simulink model "Practica1"  (R2024a)
settings: Solver=VariableStepAuto  StartTime=0.0  StopTime=10  RelTol=1e-3
InitFcn:
  | m1=0.2;
  | I1=0.3;
  | m2=0.1;
  | I2=0.25;
  | g=9.81;
settings Model: Creator=Becho  LastModifiedBy=Becho

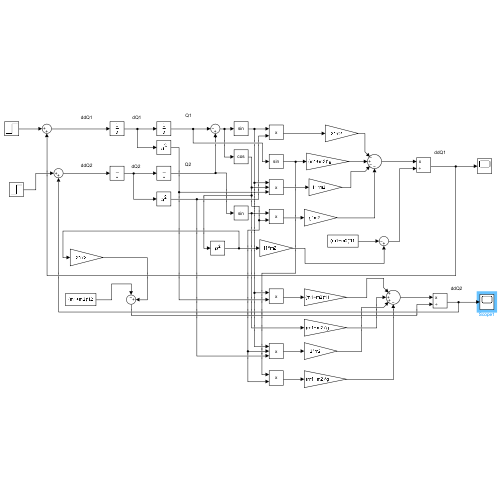
[thumbnail: Simulink's stored preview of the top-level diagram]
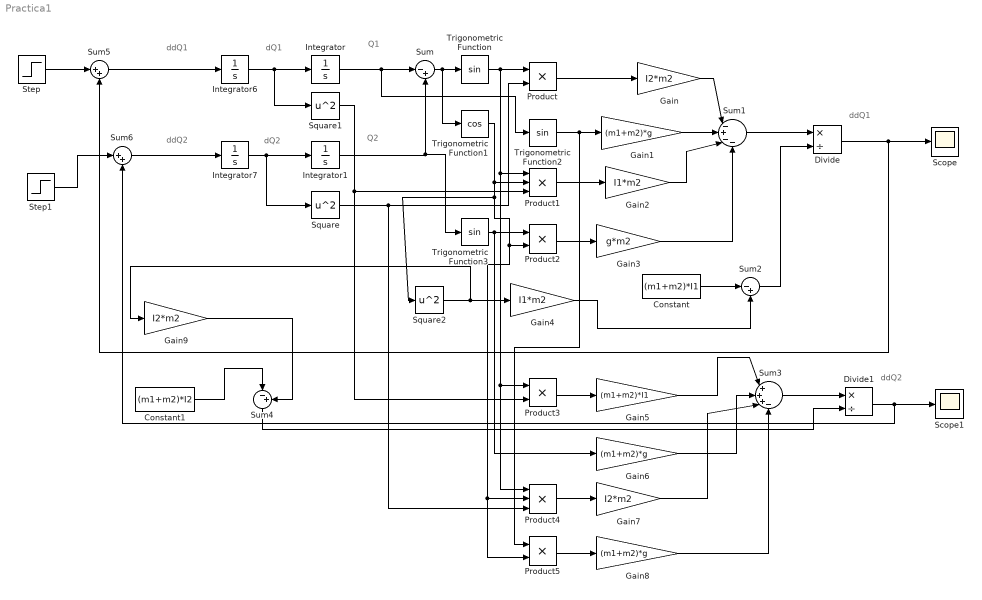
== system Practica1 ==
  note: dQ1
  note: Q2
  note: Q1
  note: dQ2
  note: ddQ1
  note: ddQ2
  note: ddQ1
  note: ddQ2
  Constant : Constant  Value=(m1+m2)*I1
  Constant1 : Constant  Value=(m1+m2)*I2
  Divide : Product  Inputs=*/
  Divide1 : Product  Inputs=*/
  Gain : Gain  Gain=I2*m2
  Gain1 : Gain  Gain=(m1+m2)*g
  Gain2 : Gain  Gain=I1*m2
  Gain3 : Gain  Gain=g*m2
  Gain4 : Gain  Gain=I1*m2
  Gain5 : Gain  Gain=(m1+m2)*I1
  Gain6 : Gain  Gain=(m1+m2)*g
  Gain7 : Gain  Gain=I2*m2
  Gain8 : Gain  Gain=(m1+m2)*g
  Gain9 : Gain  Gain=I2*m2
  Integrator : Integrator
  Integrator1 : Integrator  InitialCondition=(35*pi)/180
  Integrator6 : Integrator
  Integrator7 : Integrator
  Product{,2..3,5} (4 alike) : Product
  Product1 : Product  Inputs=3
  Product4 : Product  Inputs=3
  Scope : Scope
  Scope1 : Scope
  Square : Math  Operator=square
  Square1 : Math  Operator=square
  Square2 : Math  Operator=square
  Step : Step  Time=0  After=0  SampleTime=0
  Step1 : Step  Time=0  After=0  SampleTime=0
  Sum : Sum  Inputs=|-+
  Sum1 : Sum  Inputs=|-+--
  Sum2 : Sum  Inputs=|-+
  Sum3 : Sum  Inputs=|+++-
  Sum4 : Sum  Inputs=|-+
  Sum5 : Sum  Inputs=|++
  Sum6 : Sum  Inputs=|++
  Trigonometric Function : Trigonometry
  Trigonometric Function1 : Trigonometry  Operator=cos
  Trigonometric Function2 : Trigonometry
  Trigonometric Function3 : Trigonometry
  wires:
  Integrator/1 -> Trigonometric Function2/1, Sum/1
  Integrator1/1 -> Trigonometric Function3/1, Sum/2
  Sum/1 -> Trigonometric Function1/1, Trigonometric Function/1
  Square/1 -> Product4/3, Product/2
  Trigonometric Function/1 -> Product4/1, Product3/1, Product1/1, Product/1
  Product/1 -> Gain/1
  Gain/1 -> Sum1/1
  Trigonometric Function2/1 -> Product5/1, Gain1/1
  Gain1/1 -> Sum1/2
  Trigonometric Function1/1 -> Square2/1, Product5/2, Product4/2, Product2/2, Product1/2
  Square1/1 -> Product3/2, Product1/3
  Product1/1 -> Gain2/1
  Gain2/1 -> Sum1/3
  Trigonometric Function3/1 -> Gain6/1, Product2/1
  Product2/1 -> Gain3/1
  Gain3/1 -> Sum1/4
  Sum1/1 -> Divide/1
  Constant/1 -> Sum2/1
  Square2/1 -> Gain9/1, Gain4/1
  Gain4/1 -> Sum2/2
  Sum2/1 -> Divide/2
  Divide/1 -> Sum5/2, Scope/1
  Integrator6/1 -> Square1/1, Integrator/1
  Integrator7/1 -> Square/1, Integrator1/1
  Product3/1 -> Gain5/1
  Gain5/1 -> Sum3/1
  Gain6/1 -> Sum3/2
  Product4/1 -> Gain7/1
  Gain7/1 -> Sum3/3
  Product5/1 -> Gain8/1
  Gain8/1 -> Sum3/4
  Sum3/1 -> Divide1/1
  Constant1/1 -> Sum4/1
  Gain9/1 -> Sum4/2
  Sum4/1 -> Divide1/2
  Divide1/1 -> Sum6/2, Scope1/1
  Step/1 -> Sum5/1
  Sum5/1 -> Integrator6/1
  Step1/1 -> Sum6/1
  Sum6/1 -> Integrator7/1
